simulink model "RCAC_PID_ESC_KF_MISO"  (R2023b)
settings: Solver=FixedStepDiscrete  StartTime=0.0  StopTime=k_end  FixedStep=1  RelTol=1e-3
values from neighbouring files (symbols this model uses):
  k_jump = 3000    [run_RCAC_ESC_KF_MISO.m]    (also in run_RCAC_ESC_RLS_MISO.m; run_RCAC_ESC_fixed_Nf_KF_MISO.m; run_RCAC_PID_ESC_KF_MISO.m; run_RCAC_PID_ESC_fixed_Nf_KF_MISO.m)
  ref_val_1 = [5; 5]    [run_RCAC_ESC_KF_MISO.m]    (also in run_RCAC_ESC_RLS_MISO.m; run_RCAC_ESC_fixed_Nf_KF_MISO.m; run_RCAC_PID_ESC_KF_MISO.m; run_RCAC_PID_ESC_fixed_Nf_KF_MISO.m)
  ref_val_2 = [10; 0]    [run_RCAC_ESC_KF_MISO.m]    (also in run_RCAC_ESC_RLS_MISO.m; run_RCAC_ESC_fixed_Nf_KF_MISO.m; run_RCAC_PID_ESC_KF_MISO.m; run_RCAC_PID_ESC_fixed_Nf_KF_MISO.m)
  u_init = [0;0]    [run_RCAC_ESC_KF_MISO.m]    (also in run_RCAC_ESC_RLS_MISO.m; run_RCAC_ESC_fixed_Nf_KF_MISO.m; run_RCAC_PID_ESC_KF_MISO.m; run_RCAC_PID_ESC_fixed_Nf_KF_MISO.m)
settings Model: Creator=Juan Augusto Paredes  LastModifiedBy=Juan Augusto Paredes

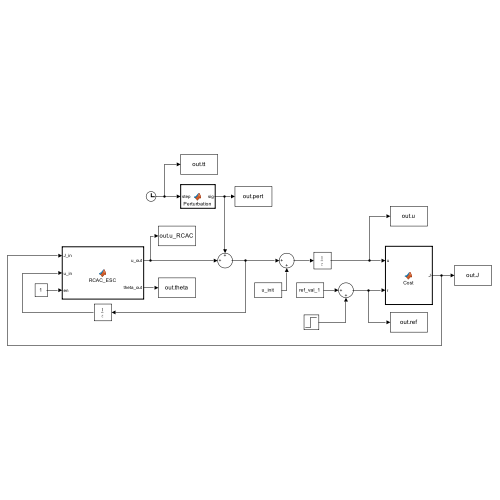
[thumbnail: Simulink's stored preview of the top-level diagram]
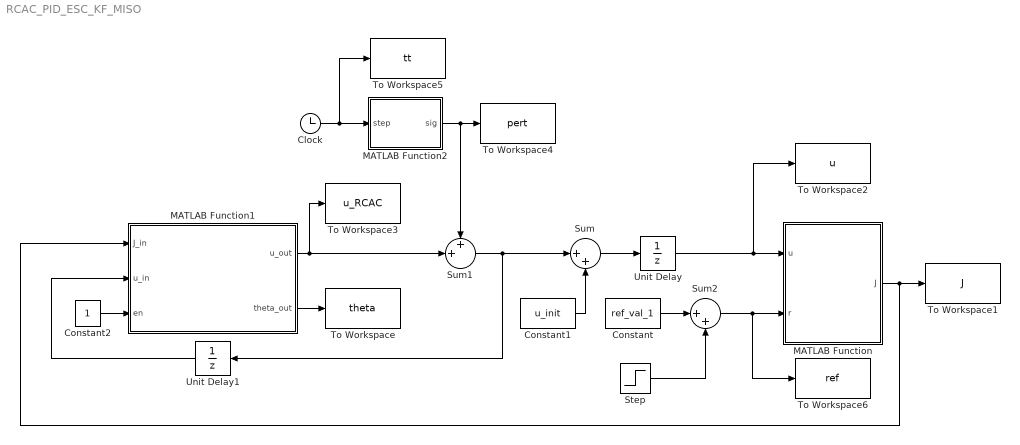
== system RCAC_PID_ESC_KF_MISO ==
  Clock : Clock
  Constant : Constant  Value=ref_val_1
  Constant1 : Constant  Value=u_init
  Constant2 : Constant
  MATLAB Function : MATLAB Function  TreatAsAtomicUnit=on
  MATLAB Function1 : MATLAB Function  TreatAsAtomicUnit=on
  MATLAB Function2 : MATLAB Function  TreatAsAtomicUnit=on
  Step : Step  Time=k_jump  After=ref_val_2-ref_val_1  SampleTime=0
  Sum : Sum  Inputs=|++
  Sum1 : Sum  Inputs=++|
  Sum2 : Sum  Inputs=|++
  To Workspace : ToWorkspace  VariableName=theta  SampleTime=-1
  To Workspace1 : ToWorkspace  VariableName=J  SampleTime=-1
  To Workspace2 : ToWorkspace  VariableName=u  SampleTime=-1
  To Workspace3 : ToWorkspace  VariableName=u_RCAC  SampleTime=-1
  To Workspace4 : ToWorkspace  VariableName=pert  SampleTime=-1
  To Workspace5 : ToWorkspace  VariableName=tt  SampleTime=-1
  To Workspace6 : ToWorkspace  VariableName=ref  SampleTime=-1
  Unit Delay : UnitDelay  InitialCondition=u_init  SampleTime=-1  HasFrameUpgradeWarning=on
  Unit Delay1 : UnitDelay  InitialCondition=[0;0]  SampleTime=-1  HasFrameUpgradeWarning=on
  wires:
  Unit Delay/1 -> To Workspace2/1, MATLAB Function/1(u)
  Sum/1 -> Unit Delay/1
  MATLAB Function1/1(u_out) -> To Workspace3/1, Sum1/2
  MATLAB Function2/1(sig) -> Sum1/1, To Workspace4/1
  Clock/1 -> To Workspace5/1, MATLAB Function2/1(step)
  Unit Delay1/1 -> MATLAB Function1/2(u_in)
  MATLAB Function/1(J) -> MATLAB Function1/1(J_in), To Workspace1/1
  MATLAB Function1/2(theta_out) -> To Workspace/1
  Constant2/1 -> MATLAB Function1/3(en)
  Sum1/1 -> Unit Delay1/1, Sum/1
  Constant1/1 -> Sum/2
  Constant/1 -> Sum2/1
  Step/1 -> Sum2/2
  Sum2/1 -> To Workspace6/1, MATLAB Function/2(r)

== matlab function RCAC_PID_ESC_KF_MISO/MATLAB Function1 ==
  settings: updateMethod=DISCRETE  sampleTime=1
  data: J_in input size=1; u_out output size=2; u_in input size=2; en input size=1; theta_out output size=40; Nc_max parameter size=1
function [u_out, theta_out] = RCAC_ESC(J_in, u_in, en, Nc_max)

persistent Grad_Est DDRCAC_PID_Cont uouttemp thetaouttemp opts

if isempty(uouttemp)
    opts = RCAC_PID_ESC_KF_MISO_define_opts();
    Grad_Est = grad_est_KF(opts.lu, opts.lz, opts.indi, opts.P0_G, opts.Q, opts.R);
    DDRCAC_PID_Cont = DDRCAC_PID(opts.lu, opts.lz, opts.PID_flag, opts.P0_C, opts.Ru, opts.nu);
    uouttemp = 0.0;
    thetaouttemp = zeros(2*Nc_max,1); 
end

theta_out = zeros(40,1); %Due to Max number for Nc = 10, can adjust by changing theta_out size

if en > 0.5
    %% Gradient estimation
    [Grad_Est, grad] = Grad_Est.oneStep(u_in, J_in, en);
    
    %% Gradient to Nf (MIMO)
    grad = grad.';
    gradNorm = sqrt(sum(grad.^2,2));
    gradNorm(gradNorm<=opts.epsi) = opts.epsi;
    Nf_temp = grad./gradNorm;
    Nf = zeros(opts.lz,opts.lu*opts.lu);
    for ii = 1:opts.lu
        Nf(:,1+(ii-1)*(opts.lu+1)) = Nf_temp(:,ii);
    end
    
    %% RCAC with Nf (DDRCAC)
    [DDRCAC_PID_Cont, uouttemp, thetaouttemp] = DDRCAC_PID_Cont.oneStep(u_in, J_in, Nf, 0);

end

u_out = uouttemp(1:2,1);
theta_out(1:2*Nc_max,1) = thetaouttemp(1:2*Nc_max,1);

end

== matlab function RCAC_PID_ESC_KF_MISO/MATLAB Function ==
  settings: updateMethod=DISCRETE
  data: u input size=2; J output size=1; r input size=2
function J = Cost(u,r)
    J = CostFcnMISO(u,r);
end

== matlab function RCAC_PID_ESC_KF_MISO/MATLAB Function2 ==
  settings: updateMethod=DISCRETE
  data: step input size=1; sig output size=2; k_jump parameter size=1
function sig = Perturbation(step, k_jump)
    sig = PertFcnMISO(step, k_jump);
end
